simulink model "Q4"  (R2017b)
settings: Solver=VariableStepAuto  StartTime=0.0  StopTime=200  RelTol=1e-3
settings Model: Creator=Kasra  LastModifiedBy=Kasra

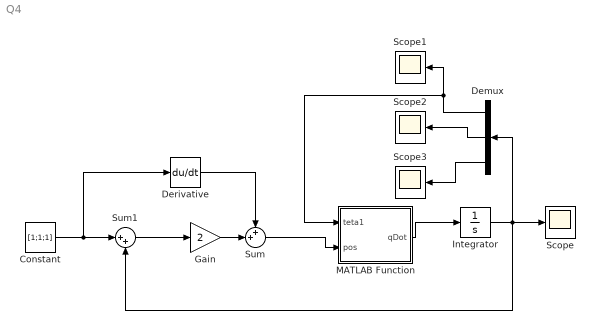
== system Q4 ==
  Constant : Constant  Value=[1;1;1]
  Demux : Demux  Outputs=3
  Derivative : Derivative
  Gain : Gain  Gain=2
  Integrator : Integrator
  MATLAB Function : MATLAB Function  TreatAsAtomicUnit=on
  Scope{,1..3} (4 alike) : Scope
  Sum : Sum  Inputs=++|
  Sum1 : Sum  Inputs=|++
  wires:
  Gain/1 -> Sum/2
  Derivative/1 -> Sum/1
  Sum/1 -> MATLAB Function/2(pos)
  Integrator/1 -> Demux/1, Sum1/2, Scope/1
  MATLAB Function/1(qDot) -> Integrator/1
  Sum1/1 -> Gain/1
  Constant/1 -> Derivative/1, Sum1/1
  Demux/1 -> MATLAB Function/1(teta1), Scope1/1
  Demux/2 -> Scope2/1
  Demux/3 -> Scope3/1

== matlab function Q4/MATLAB Function ==
  data: teta1 input; pos input; qDot output
function qDot = fcn(teta1, pos)
mat = [250*(sin(teta1)) 250*(sin(teta1)) 0; 150-250*(cos(teta1)) 250*(cos(teta1)) 0; 0 0 -1]%; 0 0 0; 0 0 0; 1 1 0];
qDot = pinv(mat) * pos;
